simulink model "SimulacionPrueba1"  (R2014b)
settings: Solver=ode45  StartTime=0.0  StopTime=10.0  RelTol=1e-3
undefined symbols (not defined in the file or in its folder): dfilt, fdesignblkfcn, gcbh
libraries: dsparch4 x2, dspsrcs4 x1
settings Model: Creator=Chehin  LastModifiedBy=Chehin

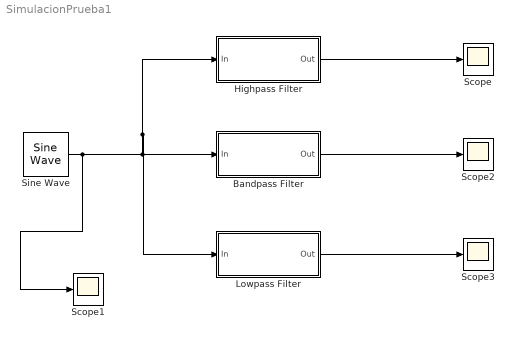
== system SimulacionPrueba1 ==
  Bandpass Filter : Subsystem  DialogController=fdesignblkfcn  InitFcn=fdesignblkfcn(gcbh, {'InitFcn'});  mask(Bandpass Filter){}
      mask help: Design a bandpass filter
      settings: CopyFcn=fdesignblkfcn(gcbh, {'CopyFcn'});
      mask Help: helpview(mapfilelocation('dsp'), 'dspbandpassfilter');
      mask Display: disp('Bandpass');
  Highpass Filter : Subsystem  DialogController=fdesignblkfcn  InitFcn=fdesignblkfcn(gcbh, {'InitFcn'});  mask(Highpass Filter){}
      mask help: Design a highpass filter
      settings: CopyFcn=fdesignblkfcn(gcbh, {'CopyFcn'});
      mask Help: helpview(mapfilelocation('dsp'), 'dsphighpassfilter');
      mask Display: disp('Highpass')
  Lowpass Filter : Subsystem  DialogController=fdesignblkfcn  InitFcn=fdesignblkfcn(gcbh, {'InitFcn'});  mask(Lowpass Filter){}
      mask help: Design a lowpass filter
      settings: CopyFcn=fdesignblkfcn(gcbh, {'CopyFcn'});
      mask Help: helpview(mapfilelocation('dsp'), 'dsplowpassfilter');
      mask Display: disp('Lowpass')
  Scope{,1..3} (4 alike) : Scope
      Scope2 settings: SaveName=ScopeData2
      Scope3 settings: SaveName=ScopeData3
  Sine Wave : dspsrcs4/Sine Wave  Amplitude=1  Frequency=150  Phase=0  SampleMode=Continuous  OutComplex=Real  CompMethod=Trigonometric fcn  TableSize=Speed  SampleTime=1/1000  SamplesPerFrame=1  ResetState=Restart at time zero  dataType=double  wordLen=16  udDataType=sfix(16)  fracBitsMode=Best precision  numFracBits=15  OutDataTypeStr=double  LastOutDataTypeStr=double
  wires:
  Sine Wave/1 -> Scope1/1, Highpass Filter/1(In), Lowpass Filter/1(In), Bandpass Filter/1(In)
  Highpass Filter/1(Out) -> Scope/1
  Bandpass Filter/1(Out) -> Scope2/1
  Lowpass Filter/1(Out) -> Scope3/1

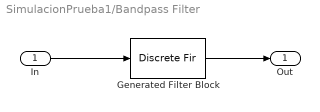
== system SimulacionPrueba1/Bandpass Filter ==
  In : Inport
  Generated Filter Block : DiscreteFir  Tag=BlockMethodSubSystem  Coefficients=[-0.020149521042045128 0.034059968047207262 0.0075914525656812643 0.024922723126907999 0.036711656123330973 -0.04895110842624488 -0.071287837277960037 0.092623520628736106 0.11310522068913756 -0.12901637626411594 -0.14173601586091997 0.14791819186205274 0.14791819186205274 -0.14173601586091997 -0.12901637626411594 0.11310522068913756 0.092623520628736106 -0.071287837277960037 -0.04895110842624488 0.036711656123330973 0.024922723126907999 0.0075914525656812643 0.034059968047207262 -0.020149521042045128]  InputProcessing=Columns as channels (frame based)
  Out : Outport
  wires:
  In/1 -> Generated Filter Block/1
  Generated Filter Block/1 -> Out/1

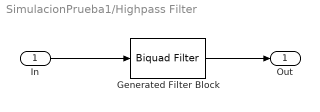
== system SimulacionPrueba1/Highpass Filter ==
  In : Inport
  Generated Filter Block : dsparch4/Biquad Filter  Tag=BlockMethodSubSystem  IIRFiltStruct=Direct form II  CoeffSource=Specify via dialog  BiQuadCoeffs=[0.15663067858621108 -0.31326135717242215 0.15663067858621108 1 0.19186656109486769 0.21295186269147323;0.60757270160483956 -1.2151454032096791 0.60757270160483956 1 -1.3497240588664159 0.91512325088943858;1 -2 1 1 -0.88766596653753482 0.67648220833345452]  a0Flag=Warning  IC=0  ICnum=0  ICden=0  InputProcessing=Columns as channels (frame based)  denAccumFracLength=30  denProdOutputFracLength=30  secondMemoryFracLength=15  roundingMode=Floor  overflowMode=off  ScaleValues=[0.76985328984737433;1;1;1.624819010617901]  optimizeScaleValues=off  ScaleValueMode=Specify via input port (g)  scaleValueFracLength=14  FilterSource=Specify via dialog  dfiltObjectName=dfilt.df2tsos([1 0.3 0.4],[1 0.1 0.2])
  Out : Outport
  wires:
  Generated Filter Block/1 -> Out/1
  In/1 -> Generated Filter Block/1

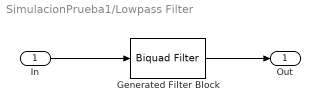
== system SimulacionPrueba1/Lowpass Filter ==
  In : Inport
  Generated Filter Block : dsparch4/Biquad Filter  Tag=BlockMethodSubSystem  IIRFiltStruct=Direct form II  CoeffSource=Specify via dialog  BiQuadCoeffs=[0.080963950232687348 0.1619279004653747 0.080963950232687348 1 -1.6956365700099822 0.74088057607053015;0.046611956969773535 0.093223913939547071 0.046611956969773535 1 -1.5640244357405921 0.92941902940892496;0.27465861782299883 0.54931723564599766 0.27465861782299883 1 -1.6097484117708694 0.81117230674854135]  a0Flag=Warning  IC=0  ICnum=0  ICden=0  InputProcessing=Columns as channels (frame based)  denAccumFracLength=30  denProdOutputFracLength=30  secondMemoryFracLength=15  roundingMode=Floor  overflowMode=off  ScaleValues=[0.044737522379358033;1;1;1]  optimizeScaleValues=off  ScaleValueMode=Specify via input port (g)  scaleValueFracLength=14  FilterSource=Specify via dialog  dfiltObjectName=dfilt.df2tsos([1 0.3 0.4],[1 0.1 0.2])
  Out : Outport
  wires:
  In/1 -> Generated Filter Block/1
  Generated Filter Block/1 -> Out/1
